simulink model "KLQR"  (R2021b)
settings: Solver=ode23t  StartTime=0.0  StopTime=inf  FixedStep=0.001  RelTol=1e-3
values from neighbouring files (symbols this model uses):
  b = 0.6    [Start.m]
  cf = -54000    [Start.m]
  cr = -54000    [Start.m]
  index_num = length(xr)    [Start.m]
  kappar = refPoses(:,5)'    [Start.m]
  m = 260    [Start.m]
  Pre_kr_num = floor(Pre_distance/d_kr)    [Start.m]
  thetar = refPoses(:,3)'    [Start.m]
  xr = refPoses(:,1)'    [Start.m]
  yr = refPoses(:,2)'    [Start.m]
libraries: vehdynlibviscommon x2, autolibshared x2, mpclib x1
settings Model: Creator=HS  LastModifiedBy=Administrator
settings SolverCC: AlgebraicLoopSolver=TrustRegion
settings OptimizationCC: DefaultParameterBehavior=Inlined  UseDivisionForNetSlopeComputation=on  GainParamInheritBuiltInType=on  UseFloatMulNetSlope=on  InlineInvariantSignals=on  PassReuseOutputArgsAs=Individual arguments  ZeroExternalMemoryAtStartup=off  ZeroInternalMemoryAtStartup=off  NoFixptDivByZeroProtection=on  EfficientFloat2IntCast=on  LifeSpan=1  OptimizeBlockOrder=speed  DifferentSizesBufferReuse=on  EfficientTunableParamExpr=on
settings DebuggingCC: ParameterTunabilityLossMsg=error  SFMachineParentedDataDiag=warning
settings HardwareCC: ProdBitPerLong=64  ProdLongLongMode=on  ProdHWDeviceType=Intel->x86-64 (Linux 64)
settings SFSimCC: MATLABDynamicMemAlloc=off
settings RTWCC: Description=Embedded Coder  SystemTargetFile=ert.tlc  GenCodeOnly=on  TemplateMakefile=ert_default_tmf  GenerateReport=on  IncludeHyperlinkInReport=on  LaunchReport=on  GenerateTraceInfo=on  GenerateTraceReport=on  GenerateTraceReportSl=on  GenerateTraceReportSf=on  GenerateTraceReportEml=on  GenerateCodeMetricsReport=on
settings CodeAppCC: ForceParamTrailComments=on  IgnoreCustomStorageClasses=off  OperatorAnnotations=on  SimulinkDataObjDesc=on  SFDataObjDesc=on  CustomSymbolStrGlobalVar=rt$N$M  CustomSymbolStrType=$N$M  CustomSymbolStrFcn=$N$M$F  CustomSymbolStrMacro=$N$M  InsertBlockDesc=on
settings ERTTargetCC: TargetLangStandard=C99 (ISO)  GenerateSampleERTMain=on  IncludeMdlTerminateFcn=off  CombineSignalStateStructs=on  SupportAbsoluteTime=off  SupportComplex=off  SupportNonInlinedSFcns=on  InlinedParameterPlacement=NonHierarchical  ERTCustomFileTemplate=example_file_process.tlc  ERTFilePackagingFormat=CompactWithDataFile

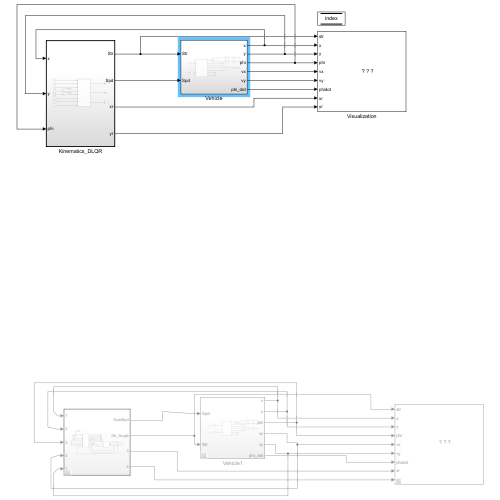
[thumbnail: Simulink's stored preview of the top-level diagram]
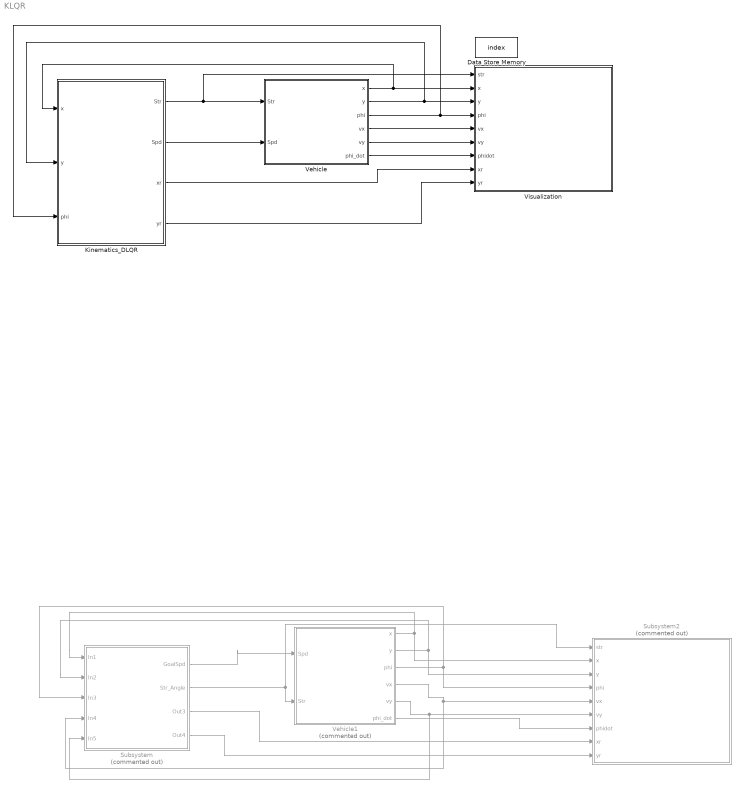
== system KLQR ==
  Data Store Memory : DataStoreMemory  DataStoreName=index  ReadBeforeWriteMsg=warning  WriteAfterWriteMsg=warning  WriteAfterReadMsg=warning  ShowAdditionalParam=off  OutDataTypeStr=double
  Kinematics_DLQR : Subsystem  TreatAsAtomicUnit=on  SystemSampleTime=0.01
  Subsystem : Subsystem  Commented=on  TreatAsAtomicUnit=on  SystemSampleTime=0.01
  Subsystem2 : Subsystem  Commented=on
      mask Display: image('C:\Users\HS\Desktop\Path_Track\Pic\visualization.JPG'); % Use "Edit Image" on toolstrip to change.
  Vehicle : Subsystem
  Vehicle1 : Subsystem  Commented=on
  Visualization : Subsystem
      mask Display: image('C:\Users\HS\Desktop\Path_Track\Pic\visualization.JPG'); % Use "Edit Image" on toolstrip to change.
  wires:
  Kinematics_DLQR/3(xr) -> Visualization/8(xr)
  Kinematics_DLQR/4(yr) -> Visualization/9(yr)
  Kinematics_DLQR/1(Str) -> Visualization/1(str), Vehicle/1(Str)
  Kinematics_DLQR/2(Spd) -> Vehicle/2(Spd)
  Vehicle/1(x) -> Kinematics_DLQR/1(x), Visualization/2(x)
  Vehicle/4(vx) -> Visualization/5(vx)
  Vehicle/5(vy) -> Visualization/6(vy)
  Vehicle/2(y) -> Visualization/3(y), Kinematics_DLQR/2(y)
  Vehicle/6(phi_dot) -> Visualization/7(phidot)
  Vehicle/3(phi) -> Visualization/4(phi), Kinematics_DLQR/3(phi)
  Vehicle1/3(phi) -> Subsystem2/4(phi), Subsystem/3(In3)
  Vehicle1/4(vx) -> Subsystem/4(In4), Subsystem2/5(vx)
  Vehicle1/5(vy) -> Subsystem/5(In5), Subsystem2/6(vy)
  Vehicle1/1(x) -> Subsystem2/2(x), Subsystem/1(In1)
  Vehicle1/2(y) -> Subsystem2/3(y), Subsystem/2(In2)
  Vehicle1/6(phi_dot) -> Subsystem2/7(phidot)
  Subsystem/2(Str_Angle) -> Subsystem2/1(str), Vehicle1/2(Str)
  Subsystem/1(GoalSpd) -> Vehicle1/1(Spd)
  Subsystem/3(Out3) -> Subsystem2/8(xr)
  Subsystem/4(Out4) -> Subsystem2/9(yr)

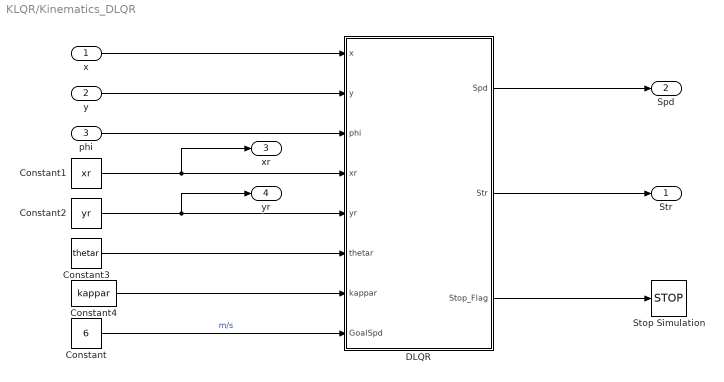
== system KLQR/Kinematics_DLQR ==
  x : Inport
  y : Inport  Port=2
  phi : Inport  Port=3
  Constant : Constant  Value=6
  Constant1 : Constant  Value=xr
  Constant2 : Constant  Value=yr
  Constant3 : Constant  Value=thetar
  Constant4 : Constant  Value=kappar
  DLQR : MATLAB Function  TreatAsAtomicUnit=on
  Stop Simulation : Stop
  Str : Outport
  Spd : Outport  Port=2
  xr : Outport  Port=3
  yr : Outport  Port=4
  wires:
  Constant2/1 -> yr/1, DLQR/5(yr)
  DLQR/3(Stop_Flag) -> Stop Simulation/1
  y/1 -> DLQR/2(y)
  Constant/1 -> DLQR/8(GoalSpd)  "m/s"
  DLQR/2(Str) -> Str/1
  Constant4/1 -> DLQR/7(kappar)
  Constant1/1 -> DLQR/4(xr), xr/1
  Constant3/1 -> DLQR/6(thetar)
  x/1 -> DLQR/1(x)
  DLQR/1(Spd) -> Spd/1
  phi/1 -> DLQR/3(phi)

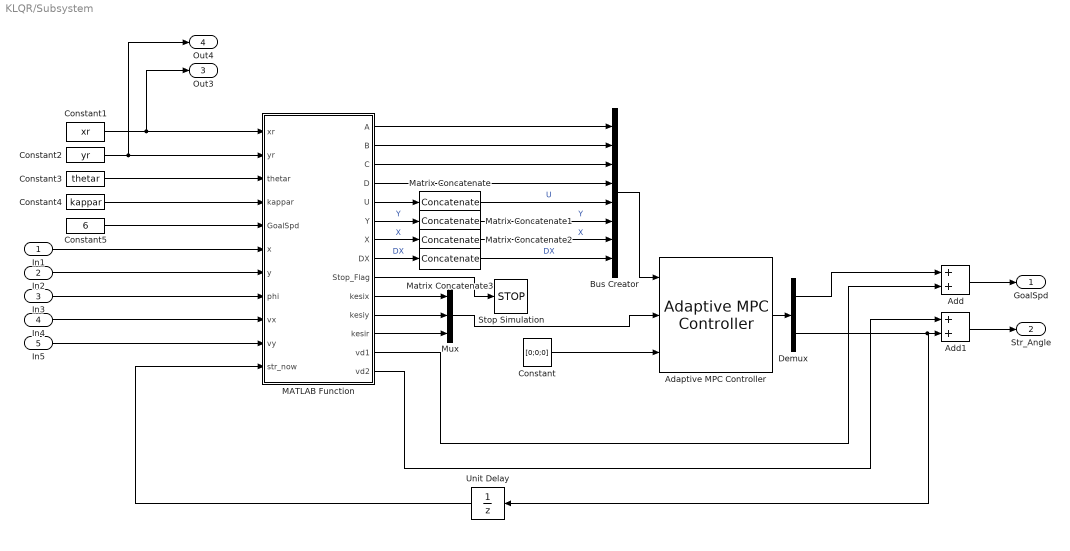
== system KLQR/Subsystem ==
  In1 : Inport
  In2 : Inport  Port=2
  In3 : Inport  Port=3
  In4 : Inport  Port=4
  In5 : Inport  Port=5
  Adaptive MPC Controller : mpclib/Adaptive MPC Controller  SCDEnableBlockLinearizationSpecification=on  mpcobj=mpcobj  enable_value=0  updateMPCinCallerWorkspace=on  md_inport=off  mv_inport=off  uref_inport=off  return_cost=off  return_mvseq=off  return_qpstatus=off  return_xseq=off  return_state=off  return_ovseq=off  state_inport=off  isltv_plant=off  umin_inport=off  umax_inport=off  ymin_inport=off  ymax_inport=off  cc_inport=off  ywt_inport=off  uwt_inport=off  duwt_inport=off  rhoeps_inport=off  pm_inport=off  MaximumP=10  HorizonChoice=FixedHorizon  BlockDataType=double  SampleTimeInherited=off  switch_inport=off
  Add : Sum
  Add1 : Sum
  Bus Creator : BusCreator  Inputs=8
  Constant : Constant  Value=[0;0;0]
  Constant1 : Constant  Value=xr
  Constant2 : Constant  Value=yr
  Constant3 : Constant  Value=thetar
  Constant4 : Constant  Value=kappar
  Constant5 : Constant  Value=6
  Demux : Demux  Outputs=2
  MATLAB Function : MATLAB Function  TreatAsAtomicUnit=on
  Matrix Concatenate : Concatenate  NumInputs=1  Mode=Multidimensional array  ConcatenateDimension=2
  Matrix Concatenate1 : Concatenate  NumInputs=1  Mode=Multidimensional array  ConcatenateDimension=3
  Matrix Concatenate2 : Concatenate  NumInputs=1  Mode=Multidimensional array  ConcatenateDimension=3
  Matrix Concatenate3 : Concatenate  NumInputs=1  Mode=Multidimensional array  ConcatenateDimension=3
  Mux : Mux  Inputs=3
  Stop Simulation : Stop
  Unit Delay : UnitDelay  SampleTime=-1  HasFrameUpgradeWarning=on
  GoalSpd : Outport
  Str_Angle : Outport  Port=2
  Out3 : Outport  Port=3
  Out4 : Outport  Port=4
  wires:
  MATLAB Function/3(C) -> Bus Creator/3
  MATLAB Function/2(B) -> Bus Creator/2
  Bus Creator/1 -> Adaptive MPC Controller/1
  MATLAB Function/4(D) -> Bus Creator/4
  MATLAB Function/1(A) -> Bus Creator/1
  Constant4/1 -> MATLAB Function/4(kappar)
  Constant/1 -> Adaptive MPC Controller/3
  Adaptive MPC Controller/1 -> Demux/1
  Constant1/1 -> Out3/1, MATLAB Function/1(xr)
  Constant3/1 -> MATLAB Function/3(thetar)
  Constant5/1 -> MATLAB Function/5(GoalSpd)
  MATLAB Function/12(kesir) -> Mux/3
  MATLAB Function/11(kesiy) -> Mux/2
  MATLAB Function/10(kesix) -> Mux/1
  Mux/1 -> Adaptive MPC Controller/2
  Constant2/1 -> Out4/1, MATLAB Function/2(yr)
  MATLAB Function/9(Stop_Flag) -> Stop Simulation/1
  Demux/1 -> Add/1
  In1/1 -> MATLAB Function/6(x)
  In2/1 -> MATLAB Function/7(y)
  In3/1 -> MATLAB Function/8(phi)
  In4/1 -> MATLAB Function/9(vx)
  In5/1 -> MATLAB Function/10(vy)
  Unit Delay/1 -> MATLAB Function/11(str_now)
  MATLAB Function/8(DX) -> Matrix Concatenate3/1  "DX"
  Add/1 -> GoalSpd/1
  Add1/1 -> Str_Angle/1
  Demux/2 -> Unit Delay/1, Add1/2
  MATLAB Function/13(vd1) -> Add/2
  MATLAB Function/14(vd2) -> Add1/1
  MATLAB Function/6(Y) -> Matrix Concatenate1/1  "Y"
  MATLAB Function/7(X) -> Matrix Concatenate2/1  "X"
  MATLAB Function/5(U) -> Matrix Concatenate/1
  Matrix Concatenate/1 -> Bus Creator/5  "U"
  Matrix Concatenate1/1 -> Bus Creator/6  "Y"
  Matrix Concatenate2/1 -> Bus Creator/7  "X"
  Matrix Concatenate3/1 -> Bus Creator/8  "DX"

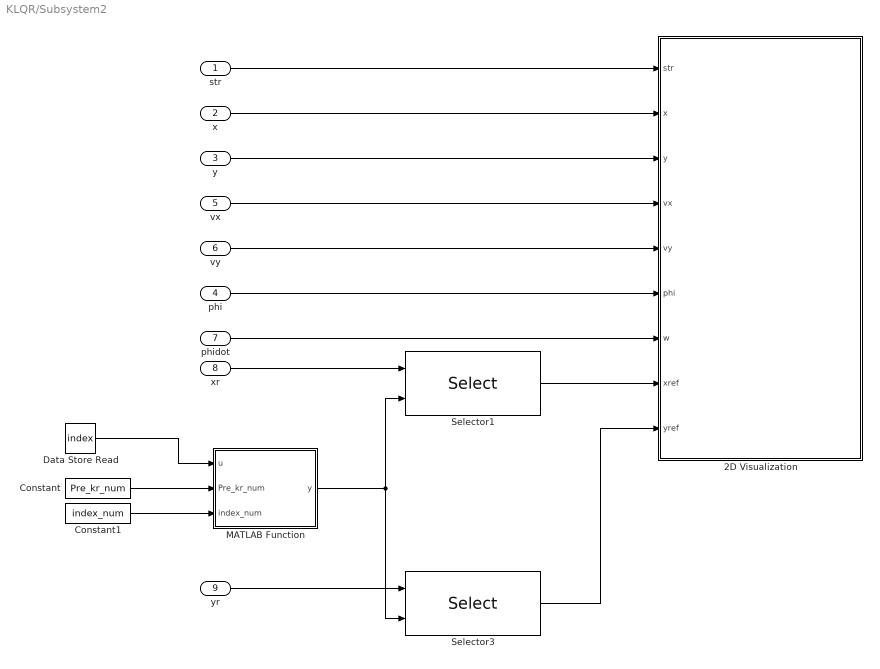
== system KLQR/Subsystem2 ==
  str : Inport
  x : Inport  Port=2
  y : Inport  Port=3
  phi : Inport  Port=4
  vx : Inport  Port=5
  vy : Inport  Port=6
  phidot : Inport  Port=7
  xr : Inport  Port=8
  yr : Inport  Port=9
  2D Visualization : Subsystem
  Constant : Constant  Value=Pre_kr_num
  Constant1 : Constant  Value=index_num
  Data Store Read : DataStoreRead  DataStoreName=index  IndexOptions=Index vector (dialog)  Indices=1  OutputSizes=1
  MATLAB Function : MATLAB Function  TreatAsAtomicUnit=on
  Selector1 : Selector  InputPortWidth=index_num  IndexOptions=Index vector (port)  Indices=[1 3]  OutputSizes=1
  Selector3 : Selector  InputPortWidth=index_num  IndexOptions=Index vector (port)  Indices=[1 3]  OutputSizes=1
  wires:
  Constant1/1 -> MATLAB Function/3(index_num)
  Constant/1 -> MATLAB Function/2(Pre_kr_num)
  MATLAB Function/1(y) -> Selector3/2, Selector1/2
  Data Store Read/1 -> MATLAB Function/1(u)
  str/1 -> 2D Visualization/1(str)
  xr/1 -> Selector1/1
  vy/1 -> 2D Visualization/5(vy)
  x/1 -> 2D Visualization/2(x)
  Selector1/1 -> 2D Visualization/8(xref)
  phidot/1 -> 2D Visualization/7(w)
  phi/1 -> 2D Visualization/6(phi)
  vx/1 -> 2D Visualization/4(vx)
  y/1 -> 2D Visualization/3(y)
  Selector3/1 -> 2D Visualization/9(yref)
  yr/1 -> Selector3/1

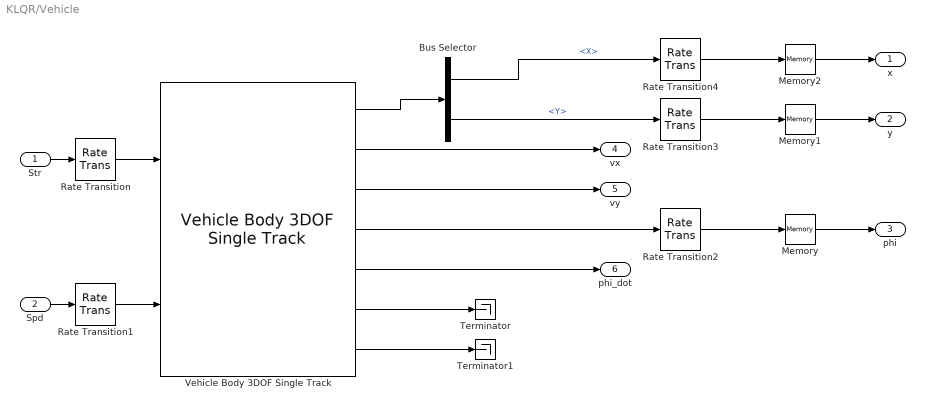
== system KLQR/Vehicle ==
  Str : Inport
  Spd : Inport  Port=2
  Bus Selector : BusSelector  OutputSignals=InertFrm.RearAxl.Disp.X,InertFrm.RearAxl.Disp.Y
  Memory : Memory
  Memory1 : Memory
  Memory2 : Memory
  Rate Transition{,1..4} (5 alike) : RateTransition
  Terminator : Terminator
  Terminator1 : Terminator
  Vehicle Body 3DOF Single Track : autolibshared/Vehicle Body 3DOF Single Track  trackMode=Single (bicycle)  inputMode=External longitudinal velocity  frontSteerMode=on  rearSteerMode=off  windMode=off  muMode=off  extFMode=off  extMMode=off  htchFMode=off  htchMMode=off  extXo=off  extpsio=off  extxdoto=off  extro=off  extYo=off  extTamb=off  extydoto=off  aMode=2  NF=2  NR=2  m=m  a=a  b=b  h=Cg_Height  dh=1  hh=0.2  X_o=xr(1)  xdot_o=0  CalphaMode=off  sigmaMode=off  d=0  hl=0  w=[1.4,1.4]  Cy_f=-cf/2  Cy_r=-cr/2  sigma_f=.1  sigma_r=.1  alpha_f_brk=[-.1 .1]  Cy_f_data=[-9e3 9e3]  alpha_r_brk=[-.1 .1]  Cy_r_data=[-9e3 9e3]  Y_o=yr(1)  ydot_o=0  Izz=Iz  psi_o=thetar(1)  r_o=0  Af=2  Cd=.3  Cl=.1  Cpm=.1  beta_w=[0:0.01:0.3]  Cs=[0:0.03:0.9]  Cym=[0:0.01:0.3]  Pabs=101325  Tair=273  g=9.81  mu=1  xdot_tol=.01  Fznom=5000  Fxtire_sat=7e4  Fytire_sat=7e4  longOff=0  latOff=0  vertOff=0  wrapAng=off
      settings: SourceProductBaseCode=PW,DR,MT,UV,VE
  x : Outport
  y : Outport  Port=2
  phi : Outport  Port=3
  vx : Outport  Port=4
  vy : Outport  Port=5
  phi_dot : Outport  Port=6
  wires:
  Vehicle Body 3DOF Single Track/1 -> Bus Selector/1
  Rate Transition1/1 -> Vehicle Body 3DOF Single Track/2
  Rate Transition4/1 -> Memory2/1
  Rate Transition/1 -> Vehicle Body 3DOF Single Track/1
  Str/1 -> Rate Transition/1
  Bus Selector/2 -> Rate Transition3/1  "<Y>"
  Rate Transition2/1 -> Memory/1
  Rate Transition3/1 -> Memory1/1
  Vehicle Body 3DOF Single Track/4 -> Rate Transition2/1
  Vehicle Body 3DOF Single Track/7 -> Terminator1/1
  Bus Selector/1 -> Rate Transition4/1  "<X>"
  Vehicle Body 3DOF Single Track/6 -> Terminator/1
  Vehicle Body 3DOF Single Track/5 -> phi_dot/1
  Vehicle Body 3DOF Single Track/2 -> vx/1
  Memory/1 -> phi/1
  Memory2/1 -> x/1
  Memory1/1 -> y/1
  Spd/1 -> Rate Transition1/1
  Vehicle Body 3DOF Single Track/3 -> vy/1

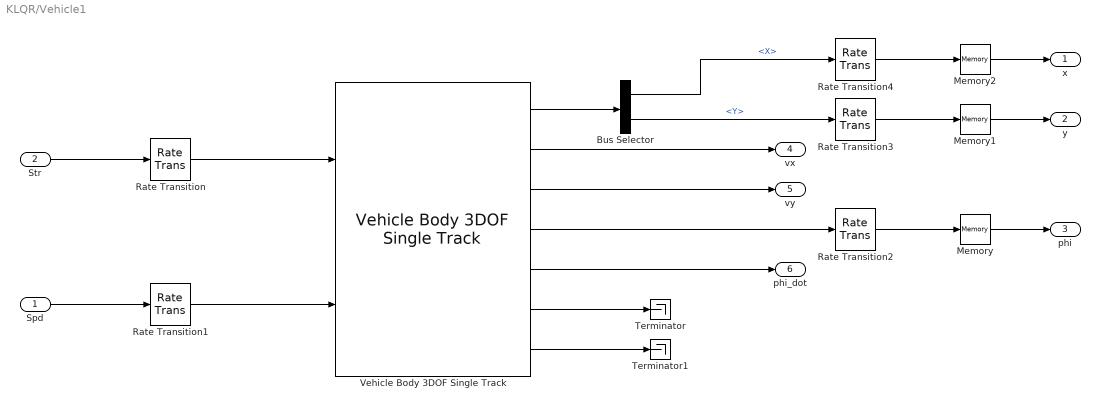
== system KLQR/Vehicle1 ==
  Spd : Inport
  Str : Inport  Port=2
  Bus Selector : BusSelector  OutputSignals=InertFrm.RearAxl.Disp.X,InertFrm.RearAxl.Disp.Y
  Memory : Memory
  Memory1 : Memory
  Memory2 : Memory
  Rate Transition{,1..4} (5 alike) : RateTransition
  Terminator : Terminator
  Terminator1 : Terminator
  Vehicle Body 3DOF Single Track : autolibshared/Vehicle Body 3DOF Single Track  trackMode=Single (bicycle)  inputMode=External longitudinal velocity  frontSteerMode=on  rearSteerMode=off  windMode=off  muMode=off  extFMode=off  extMMode=off  extXo=off  extpsio=off  extxdoto=off  extro=off  extYo=off  extTamb=off  extydoto=off  aMode=2  NF=2  NR=2  m=m  a=a  b=b  h=Cg_Height  X_o=xr(1)  xdot_o=0  CalphaMode=off  sigmaMode=off  d=0  w=[1.4,1.4]  Cy_f=-cf/2  Cy_r=-cr/2  sigma_f=.1  sigma_r=.1  alpha_f_brk=[-.1 .1]  Cy_f_data=[-9e3 9e3]  alpha_r_brk=[-.1 .1]  Cy_r_data=[-9e3 9e3]  Y_o=yr(1)  ydot_o=0  Izz=Iz  psi_o=thetar(1)  r_o=0  Af=2  Cd=.3  Cl=.1  Cpm=.1  beta_w=[0:0.01:0.3]  Cs=[0:0.03:0.9]  Cym=[0:0.01:0.3]  Pabs=101325  Tair=273  g=9.81  mu=1  xdot_tol=.01  Fznom=5000  Fxtire_sat=7e4  Fytire_sat=7e4  longOff=0  latOff=0  vertOff=0  wrapAng=off
      settings: SourceProductBaseCode=PW,DR,MT,UV,VE
  x : Outport
  y : Outport  Port=2
  phi : Outport  Port=3
  vx : Outport  Port=4
  vy : Outport  Port=5
  phi_dot : Outport  Port=6
  wires:
  Vehicle Body 3DOF Single Track/1 -> Bus Selector/1
  Rate Transition1/1 -> Vehicle Body 3DOF Single Track/2
  Rate Transition4/1 -> Memory2/1
  Rate Transition/1 -> Vehicle Body 3DOF Single Track/1
  Str/1 -> Rate Transition/1
  Bus Selector/2 -> Rate Transition3/1  "<Y>"
  Rate Transition2/1 -> Memory/1
  Rate Transition3/1 -> Memory1/1
  Vehicle Body 3DOF Single Track/4 -> Rate Transition2/1
  Vehicle Body 3DOF Single Track/7 -> Terminator1/1
  Bus Selector/1 -> Rate Transition4/1  "<X>"
  Vehicle Body 3DOF Single Track/6 -> Terminator/1
  Vehicle Body 3DOF Single Track/5 -> phi_dot/1
  Vehicle Body 3DOF Single Track/2 -> vx/1
  Memory/1 -> phi/1
  Memory2/1 -> x/1
  Memory1/1 -> y/1
  Spd/1 -> Rate Transition1/1
  Vehicle Body 3DOF Single Track/3 -> vy/1

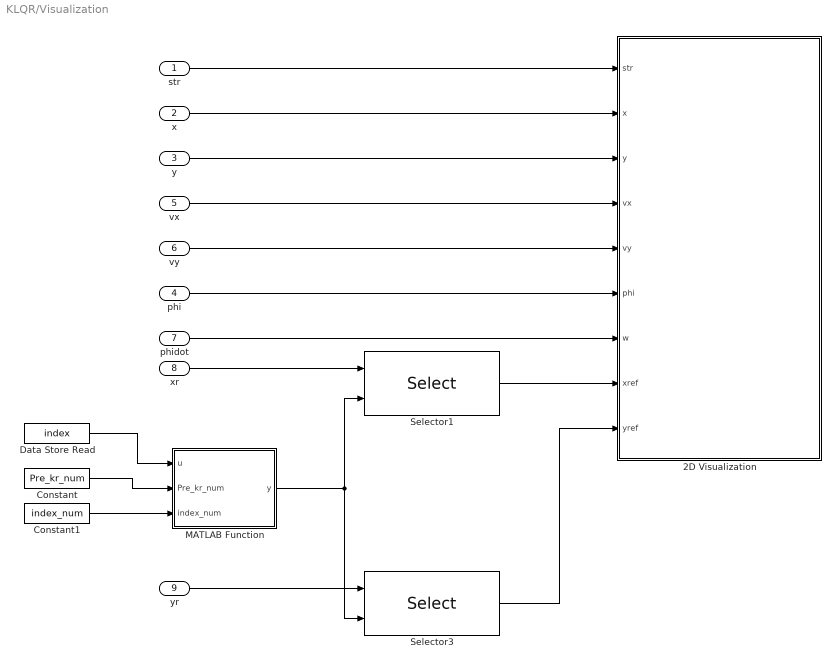
== system KLQR/Visualization ==
  str : Inport
  x : Inport  Port=2
  y : Inport  Port=3
  phi : Inport  Port=4
  vx : Inport  Port=5
  vy : Inport  Port=6
  phidot : Inport  Port=7
  xr : Inport  Port=8
  yr : Inport  Port=9
  2D Visualization : Subsystem
  Constant : Constant  Value=Pre_kr_num
  Constant1 : Constant  Value=index_num
  Data Store Read : DataStoreRead  DataStoreName=index  IndexOptions=Index vector (dialog)  Indices=1  OutputSizes=1
  MATLAB Function : MATLAB Function  TreatAsAtomicUnit=on
  Selector1 : Selector  InputPortWidth=index_num  IndexOptions=Index vector (port)  Indices=[1 3]  OutputSizes=1
  Selector3 : Selector  InputPortWidth=index_num  IndexOptions=Index vector (port)  Indices=[1 3]  OutputSizes=1
  wires:
  yr/1 -> Selector3/1
  Selector3/1 -> 2D Visualization/9(yref)
  y/1 -> 2D Visualization/3(y)
  vx/1 -> 2D Visualization/4(vx)
  phi/1 -> 2D Visualization/6(phi)
  phidot/1 -> 2D Visualization/7(w)
  Selector1/1 -> 2D Visualization/8(xref)
  x/1 -> 2D Visualization/2(x)
  vy/1 -> 2D Visualization/5(vy)
  xr/1 -> Selector1/1
  str/1 -> 2D Visualization/1(str)
  Data Store Read/1 -> MATLAB Function/1(u)
  MATLAB Function/1(y) -> Selector1/2, Selector3/2
  Constant/1 -> MATLAB Function/2(Pre_kr_num)
  Constant1/1 -> MATLAB Function/3(index_num)

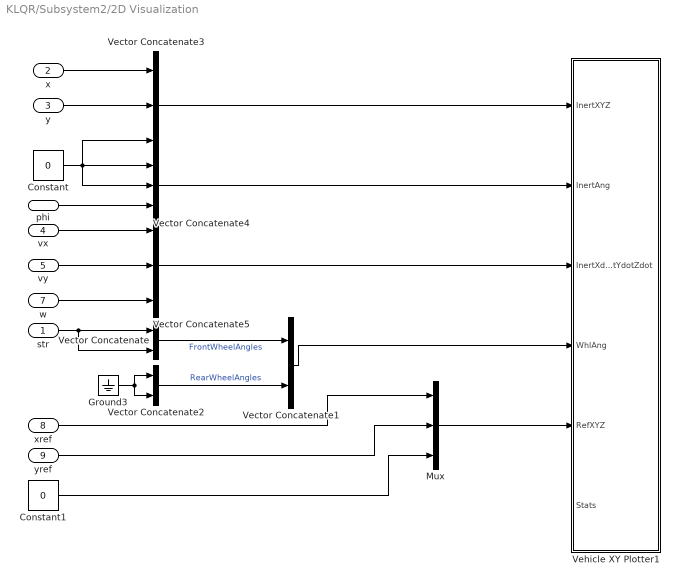
== system KLQR/Subsystem2/2D Visualization ==
  str : Inport
  x : Inport  Port=2
  y : Inport  Port=3
  vx : Inport  Port=4
  vy : Inport  Port=5
  phi : Inport  Port=6
  w : Inport  Port=7
  xref : Inport  Port=8
  yref : Inport  Port=9
  Constant : Constant  Value=0
  Constant1 : Constant  Value=0
  Ground3 : Ground
  Mux : Mux  Inputs=3
  Vector Concatenate : Concatenate
  Vector Concatenate1 : Concatenate
  Vector Concatenate2 : Concatenate
  Vector Concatenate3 : Concatenate  NumInputs=3
  Vector Concatenate4 : Concatenate  NumInputs=3
  Vector Concatenate5 : Concatenate  NumInputs=3
  Vehicle XY Plotter1 : Subsystem  mask(Vehicle XY Plotter){extRef=on, extStats=on, extTireF=off, a=1, b=0.6, w=1.49, figBorder=20, bufferSize=1024, velNorm=2, tireFNorm=1000, pltDT=0.05}
      mask prompts: extRef "Plot path reference, extRef"; extStats "Display speed, RPM and Gear"; extTireF "Display tire forces"; a "Distance to front axle from CG, a [m]:"; b "Distance to rear axle from CG, b [m]:"; w "Track width, w [m]:"; figBorder "Distance to figure borders, figBorder [m]:"; bufferSize "Path buffer sampe size, bufferSize []:"; velNorm "Velocity vector scaling, velNorm [m*s/m]:"; tireFNorm "Tire force vector scaling, tireFNorm [m/N]:"; pltDT "Plot update rate, pltDT [s]:"
      mask help:
      | This block will display a MATLAB figure which indicates the vehicle path, current position and heading velocity.
      | An optional path reference is also provided.
      mask init:
      | block = gcb;
      | if autoblkschecksimstopped(block)
      |     ParamNames = {'extRef';'extStats';'extTireF';'extTireF'};
      |     PortNames = {'RefXYZ';'Stats';'TireFx';'TireFy'};
      |     for idx=1:length(PortNames)
      |         InportOption  = {'built-in/Ground', [PortNames{idx}, ' Ground'];...
      |             'built-in/Inport',PortNames{idx}};
      |         if ~strcmp(get_param(block,ParamNames{idx}),'on')
      |             NewBlkHdl = autoblksreplaceblock(block, InportOption, 1);
      |             set_param(NewBlkHdl, 'ShowName', 'off');
      |         else
      |             autoblksreplaceblock(block, InportOption, 2);
      |         end
      |     end
      |     InportNames = {'InertXYZ';'InertAng';'InertXdotYdotZdot';'WhlAng';'RefXYZ';'Stats';'TireFx';'TireFy'};
      |     FoundNames = get_param(find_system(block, 'LookUnderMasks', 'all', 'SearchDepth', 1, 'FollowLinks', 'on', 'BlockType', 'Inport'), 'Name');
      |     [~,PortI] = intersect(InportNames, FoundNames);
      |     PortI = sort(PortI);
      |     for idx = 1:length(PortI)
      |         set_param([block, '/', InportNames{PortI(idx)}], 'Port', num2str(idx));
      |     end
      | end
      mask TypeOptions a: Vehicle XY Plotter/a
      mask TypeOptions b: Vehicle XY Plotter/b
      mask TypeOptions w: Vehicle XY Plotter/w
      mask TypeOptions figBorder: Vehicle XY Plotter/figBorder
      mask TypeOptions bufferSize: Vehicle XY Plotter/bufferSize
      mask TypeOptions velNorm: Vehicle XY Plotter/velNorm
      mask TypeOptions tireFNorm: Vehicle XY Plotter/tireFNorm
      mask DialogControl Container3 Prompt: Plot and Display Options
  wires:
  phi/1 -> Vector Concatenate4/3
  Constant1/1 -> Mux/3
  yref/1 -> Mux/2
  xref/1 -> Mux/1
  Mux/1 -> Vehicle XY Plotter1/5(RefXYZ)
  str/1 -> Vector Concatenate/1, Vector Concatenate/2
  vx/1 -> Vector Concatenate5/1
  w/1 -> Vector Concatenate5/3
  vy/1 -> Vector Concatenate5/2
  Constant/1 -> Vector Concatenate4/2, Vector Concatenate4/1, Vector Concatenate3/3
  y/1 -> Vector Concatenate3/2
  x/1 -> Vector Concatenate3/1
  Vector Concatenate4/1 -> Vehicle XY Plotter1/2(InertAng)
  Vector Concatenate3/1 -> Vehicle XY Plotter1/1(InertXYZ)
  Vector Concatenate5/1 -> Vehicle XY Plotter1/3(InertXdotYdotZdot)
  Vector Concatenate2/1 -> Vector Concatenate1/2  "RearWheelAngles"
  Vector Concatenate/1 -> Vector Concatenate1/1  "FrontWheelAngles"
  Ground3/1 -> Vector Concatenate2/2, Vector Concatenate2/1
  Vector Concatenate1/1 -> Vehicle XY Plotter1/4(WhlAng)

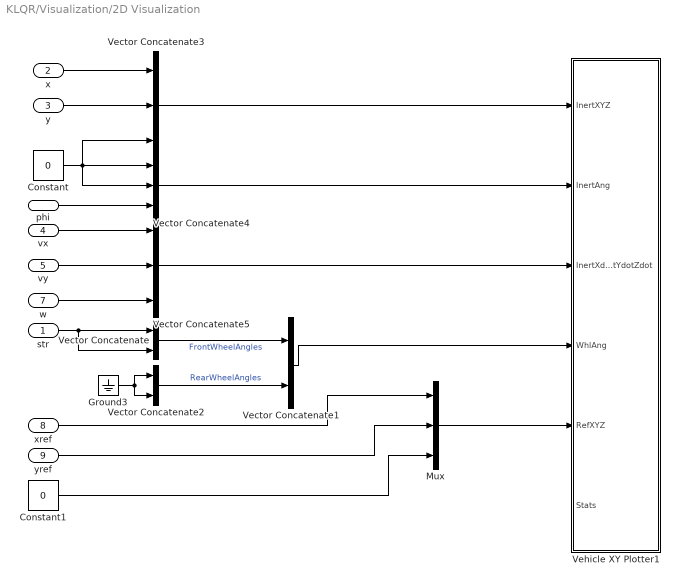
== system KLQR/Visualization/2D Visualization ==
  str : Inport
  x : Inport  Port=2
  y : Inport  Port=3
  vx : Inport  Port=4
  vy : Inport  Port=5
  phi : Inport  Port=6
  w : Inport  Port=7
  xref : Inport  Port=8
  yref : Inport  Port=9
  Constant : Constant  Value=0
  Constant1 : Constant  Value=0
  Ground3 : Ground
  Mux : Mux  Inputs=3
  Vector Concatenate : Concatenate
  Vector Concatenate1 : Concatenate
  Vector Concatenate2 : Concatenate
  Vector Concatenate3 : Concatenate  NumInputs=3
  Vector Concatenate4 : Concatenate  NumInputs=3
  Vector Concatenate5 : Concatenate  NumInputs=3
  Vehicle XY Plotter1 : Subsystem  mask(Vehicle XY Plotter){extRef=on, extStats=on, extTireF=off, a=1, b=0.6, w=1.49, figBorder=20, bufferSize=1024, velNorm=2, tireFNorm=1000, pltDT=0.05}
      mask prompts: extRef "Plot path reference, extRef"; extStats "Display speed, RPM and Gear"; extTireF "Display tire forces"; a "Distance to front axle from CG, a [m]:"; b "Distance to rear axle from CG, b [m]:"; w "Track width, w [m]:"; figBorder "Distance to figure borders, figBorder [m]:"; bufferSize "Path buffer sampe size, bufferSize []:"; velNorm "Velocity vector scaling, velNorm [m*s/m]:"; tireFNorm "Tire force vector scaling, tireFNorm [m/N]:"; pltDT "Plot update rate, pltDT [s]:"
      mask help:
      | This block will display a MATLAB figure which indicates the vehicle path, current position and heading velocity.
      | An optional path reference is also provided.
      mask init: same as KLQR/Subsystem2/2D Visualization/Vehicle XY Plotter1
      mask TypeOptions a: Vehicle XY Plotter/a
      mask TypeOptions b: Vehicle XY Plotter/b
      mask TypeOptions w: Vehicle XY Plotter/w
      mask TypeOptions figBorder: Vehicle XY Plotter/figBorder
      mask TypeOptions bufferSize: Vehicle XY Plotter/bufferSize
      mask TypeOptions velNorm: Vehicle XY Plotter/velNorm
      mask TypeOptions tireFNorm: Vehicle XY Plotter/tireFNorm
      mask DialogControl Container3 Prompt: Plot and Display Options
  wires:
  Vector Concatenate1/1 -> Vehicle XY Plotter1/4(WhlAng)
  Ground3/1 -> Vector Concatenate2/1, Vector Concatenate2/2
  Vector Concatenate/1 -> Vector Concatenate1/1  "FrontWheelAngles"
  Vector Concatenate2/1 -> Vector Concatenate1/2  "RearWheelAngles"
  Vector Concatenate5/1 -> Vehicle XY Plotter1/3(InertXdotYdotZdot)
  Vector Concatenate3/1 -> Vehicle XY Plotter1/1(InertXYZ)
  Vector Concatenate4/1 -> Vehicle XY Plotter1/2(InertAng)
  x/1 -> Vector Concatenate3/1
  y/1 -> Vector Concatenate3/2
  Constant/1 -> Vector Concatenate3/3, Vector Concatenate4/1, Vector Concatenate4/2
  vy/1 -> Vector Concatenate5/2
  w/1 -> Vector Concatenate5/3
  vx/1 -> Vector Concatenate5/1
  str/1 -> Vector Concatenate/2, Vector Concatenate/1
  Mux/1 -> Vehicle XY Plotter1/5(RefXYZ)
  xref/1 -> Mux/1
  yref/1 -> Mux/2
  Constant1/1 -> Mux/3
  phi/1 -> Vector Concatenate4/3

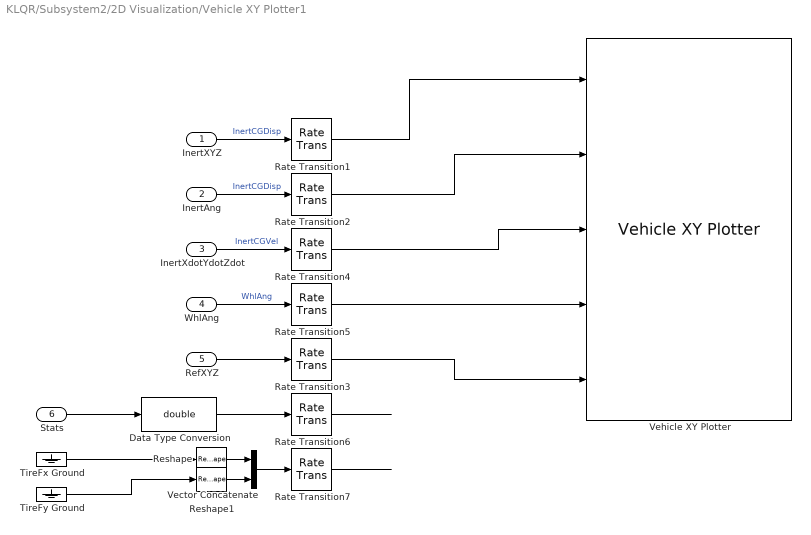
== system KLQR/Subsystem2/2D Visualization/Vehicle XY Plotter1 ==
  InertXYZ : Inport
  InertAng : Inport  Port=2
  InertXdotYdotZdot : Inport  Port=3
  WhlAng : Inport  Port=4
  RefXYZ : Inport  Port=5
  Stats : Inport  Port=6
  Data Type Conversion : DataTypeConversion  OutDataTypeStr=double
  Rate Transition{1..7} (7 alike) : RateTransition  Deterministic=off  OutPortSampleTime=pltDT
  Reshape : Reshape  OutputDimensionality=Row vector (2-D)
  Reshape1 : Reshape  OutputDimensionality=Row vector (2-D)
  TireFx Ground : Ground
  TireFy Ground : Ground
  Vector Concatenate : Concatenate  Mode=Multidimensional array
  Vehicle XY Plotter : vehdynlibviscommon/Vehicle XY Plotter  w=w  a=a  b=b  figBorder=figBorder  bufferSize=bufferSize  extStats=off  extTireF=off
      settings: SourceProductBaseCode=VE
  wires:
  Stats/1 -> Data Type Conversion/1
  TireFy Ground/1 -> Reshape1/1
  TireFx Ground/1 -> Reshape/1
  InertAng/1 -> Rate Transition2/1  "InertCGDisp"
  InertXdotYdotZdot/1 -> Rate Transition4/1  "InertCGVel"
  InertXYZ/1 -> Rate Transition1/1  "InertCGDisp"
  WhlAng/1 -> Rate Transition5/1  "WhlAng"
  Rate Transition3/1 -> Vehicle XY Plotter/5
  Rate Transition1/1 -> Vehicle XY Plotter/1
  Rate Transition2/1 -> Vehicle XY Plotter/2
  Rate Transition4/1 -> Vehicle XY Plotter/3
  Rate Transition5/1 -> Vehicle XY Plotter/4
  Rate Transition6/1 -> ?
  Data Type Conversion/1 -> Rate Transition6/1
  Rate Transition7/1 -> ?
  RefXYZ/1 -> Rate Transition3/1
  Reshape/1 -> Vector Concatenate/1
  Reshape1/1 -> Vector Concatenate/2
  Vector Concatenate/1 -> Rate Transition7/1

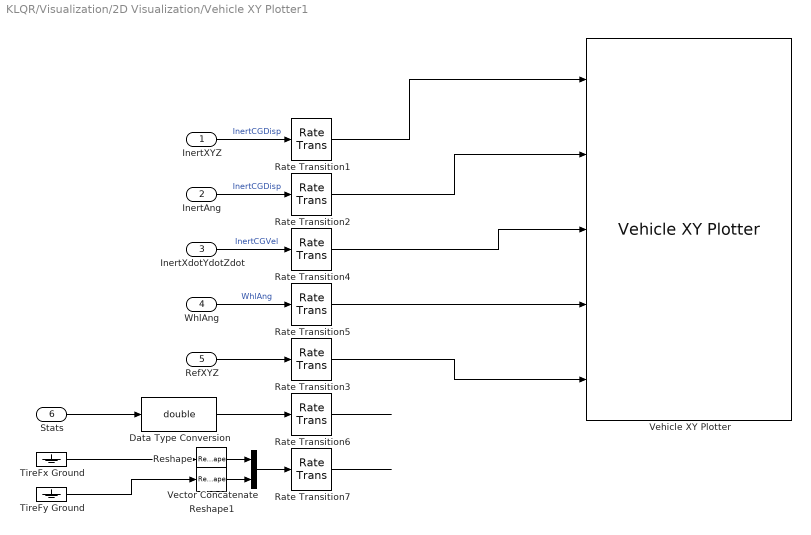
== system KLQR/Visualization/2D Visualization/Vehicle XY Plotter1 ==
  InertXYZ : Inport
  InertAng : Inport  Port=2
  InertXdotYdotZdot : Inport  Port=3
  WhlAng : Inport  Port=4
  RefXYZ : Inport  Port=5
  Stats : Inport  Port=6
  Data Type Conversion : DataTypeConversion  OutDataTypeStr=double
  Rate Transition{1..7} (7 alike) : RateTransition  Deterministic=off  OutPortSampleTime=pltDT
  Reshape : Reshape  OutputDimensionality=Row vector (2-D)
  Reshape1 : Reshape  OutputDimensionality=Row vector (2-D)
  TireFx Ground : Ground
  TireFy Ground : Ground
  Vector Concatenate : Concatenate  Mode=Multidimensional array
  Vehicle XY Plotter : vehdynlibviscommon/Vehicle XY Plotter  w=w  a=a  b=b  figBorder=figBorder  bufferSize=bufferSize  extStats=off  extTireF=off
      settings: SourceProductBaseCode=VE
  wires:
  Vector Concatenate/1 -> Rate Transition7/1
  Reshape1/1 -> Vector Concatenate/2
  Reshape/1 -> Vector Concatenate/1
  RefXYZ/1 -> Rate Transition3/1
  Rate Transition7/1 -> ?
  Data Type Conversion/1 -> Rate Transition6/1
  Rate Transition6/1 -> ?
  Rate Transition5/1 -> Vehicle XY Plotter/4
  Rate Transition4/1 -> Vehicle XY Plotter/3
  Rate Transition2/1 -> Vehicle XY Plotter/2
  Rate Transition1/1 -> Vehicle XY Plotter/1
  Rate Transition3/1 -> Vehicle XY Plotter/5
  WhlAng/1 -> Rate Transition5/1  "WhlAng"
  InertXYZ/1 -> Rate Transition1/1  "InertCGDisp"
  InertXdotYdotZdot/1 -> Rate Transition4/1  "InertCGVel"
  InertAng/1 -> Rate Transition2/1  "InertCGDisp"
  TireFx Ground/1 -> Reshape/1
  TireFy Ground/1 -> Reshape1/1
  Stats/1 -> Data Type Conversion/1

== matlab function KLQR/Subsystem2/MATLAB Function ==
  data: u input; Pre_kr_num input; index_num input; y output
function y = fcn(u, Pre_kr_num, index_num)

if u + Pre_kr_num*8 < index_num
    y = u + Pre_kr_num*8;
else
    y = index_num;
end

end

== matlab function KLQR/Subsystem/MATLAB Function ==
  data: xr input; A output; yr input; thetar input; kappar input; GoalSpd input; x input; y input; phi input; vx input; vy input; str_now input; B output; C output; D output; U output; Y output; X output; DX output; Stop_Flag output; kesix output; kesiy output; kesir output; index data_store_memory; vd1 output; vd2 output
function [A,B,C,D,U,Y,X,DX,Stop_Flag,kesix,kesiy,kesir,vd1,vd2] = fcn(xr,yr,thetar,kappar,GoalSpd,x,y,phi,vx,vy,str_now)
%****初始化参数矩阵************%
global index;
T = 0.01;%程序离散控制周期，配合原子子系统0.01ms周期
L = 1.6;%车辆轴距
n=length(xr);      %路径点个数
Stop_Flag = 0;     %仿真结束标志位
%coder.extrinsic('dlqr'); %若用自带库函数，请用外部声明
min=1;
%*******寻找车辆后轴与当前车辆最近点，仅查找距上一次车辆位置最近点前30个点
    if index == 0  %%Code has not run yet;
		d_min=(x-xr(1))^2+(y-yr(1))^2;
		min=1;
		for i=1:30 %% search 1-30 points when car is running.
			d=(x-xr(i))^2+(y-yr(i))^2;
			if d<d_min
				d_min=d;
				min=i;
			end
		end
		dmin=min;
		index = dmin; %% dmin assigns to index;
    else
		d_min = (x-xr(index))^2+(y-yr(index))^2;
		min = index;
		if index <= n - 30
			for i = index:index+30
				d=(x-xr(i))^2+(y-yr(i))^2;
				if d<d_min
					d_min=d;
					min=i;
				end
			end
			dmin=min;
			index = dmin;
		else 
			for i = index:n
				d=(x-xr(i))^2+(y-yr(i))^2;
				if d<d_min
					d_min=d;
					min=i;
                    if min == n
                        Stop_Flag =1;%路径点跑完了仿真停止
                    end
				end
			end
			dmin=min;
			index = dmin; 
		end
    end
%*****状态变量计算******%
kesix = x -xr(dmin);
kesiy = y -yr(dmin);
kesir =phi - thetar(dmin);
  %******防止数据溢出***********%
    if kesir < -3.14
        kesir = kesir+6.28;
    end
    if kesir >3.14
        kesir = kesir -6.28;
    end
xstate = [kesix;
          kesiy;
          kesir];%状态变量
vd1 = GoalSpd; %期望速度
t_d = thetar(dmin);%当前和车辆最近点的航向角
k = kappar(dmin);%当前和车辆最近点的曲率
vd2=atan(L*k);%期望前轮转角
Ad=[1    0   -vd1*sin(t_d)*T;
    0    1   vd1*cos(t_d)*T;
    0    0    1;];  %线性离散后的系统矩阵   
Bd=[cos(t_d)*T     0;
    sin(t_d)*T     0;
    tan(vd2)*T/L   vd1*T/(L*(cos(vd2)^2))]; %线性离散后的控制矩阵
Cd =[1 0 0;
    0 1 0;
    0 0 1;];
Dd = [0 0 ; 0  0;0  0];
A =Ad;
B =Bd;
C =Cd;
D =Dd;
X = xstate;
v_now =sqrt(vx^2+vy^2);
U = [vd1 - v_now;
    vd2 - str_now];
Y =C*xstate;
DX = A*xstate+B*U-xstate;





end

== matlab function KLQR/Visualization/MATLAB Function ==
  data: u input; Pre_kr_num input; index_num input; y output
function y = fcn(u, Pre_kr_num, index_num)

if u + Pre_kr_num*8 < index_num
    y = u + Pre_kr_num*8;
else
    y = index_num;
end

end

== matlab function KLQR/Kinematics_DLQR/DLQR ==
  settings: updateMethod=DISCRETE
  data: Spd output; Str output; x input; y input; phi input; xr input; yr input; thetar input; kappar input; Stop_Flag output; index data_store_memory; GoalSpd input

function [Spd,Str,Stop_Flag]  = fcn(x,y,phi,xr,yr,thetar,kappar,GoalSpd)
%****初始化参数矩阵************%
global index;
T = 0.01;%程序离散控制周期，配合原子子系统0.01ms周期
L = 1.6;%车辆轴距
PN_1 = zeros(3,3); %该矩阵用于黎卡提方程迭代
n=length(xr);      %路径点个数
Stop_Flag = 0;     %仿真结束标志位
I = eye(3);        %初始化3*3单位矩阵
K =zeros(2,3);     %初始化反馈增益矩阵维度
%coder.extrinsic('dlqr'); %若用自带库函数，请用外部声明
min=1;
%*******寻找车辆后轴与当前车辆最近点，仅查找距上一次车辆位置最近点前30个点
    if index == 0  %%Code has not run yet;
		d_min=(x-xr(1))^2+(y-yr(1))^2;
		min=1;
		for i=1:30 %% search 1-30 points when car is running.
			d=(x-xr(i))^2+(y-yr(i))^2;
			if d<d_min
				d_min=d;
				min=i;
			end
		end
		dmin=min;
		index = dmin; %% dmin assigns to index;
    else
		d_min = (x-xr(index))^2+(y-yr(index))^2;
		min = index;
		if index <= n - 30
			for i = index:index+30
				d=(x-xr(i))^2+(y-yr(i))^2;
				if d<d_min
					d_min=d;
					min=i;
				end
			end
			dmin=min;
			index = dmin;
		else 
			for i = index:n
				d=(x-xr(i))^2+(y-yr(i))^2;
				if d<d_min
					d_min=d;
					min=i;
                    if min == n
                        Stop_Flag =1;%路径点跑完了仿真停止
                    end
				end
			end
			dmin=min;
			index = dmin; 
		end
    end
%*****状态变量计算******%
kesix = x -xr(dmin);
kesiy = y -yr(dmin);
kesir =phi - thetar(dmin);
  %******防止偏差数据溢出***********%
    if kesir < -3.14
        kesir = kesir+6.28;
    end
    if kesir >3.14
        kesir = kesir -6.28;
    end

xstate = [kesix;
          kesiy;
          kesir];%状态变量
vd1 = GoalSpd; %期望速度
t_d = thetar(dmin);%当前和车辆最近点的航向角
k = kappar(dmin);%当前和车辆最近点的曲率
vd2=atan(L*k);%期望前轮转角

Ad=[1    0   -vd1*sin(t_d)*T;
    0    1   vd1*cos(t_d)*T;
    0    0    1;];  %线性离散后的系统矩阵
   
Bd=[cos(t_d)*T     0;
    sin(t_d)*T     0;
    tan(vd2)*T/L   vd1*T/(L*(cos(vd2)^2))]; %线性离散后的控制矩阵
   
 Q = [10 0 0;
      0 10 0; 
      0 0 10];%初始化LQR的权重矩阵
 R =[5 0;
     0 5];%初始化LQR的权重矩阵
 
 %*********黎卡提方程求解**********%
 PN =Q;  
 err =10^(-1);%该精度根据需要调整，误差越小迭代次数越多
 error = 1;
 while(error>err)
        PN_1 = Q+Ad'*PN/(I+Bd/R*Bd'*PN)*Ad;%黎卡提方程
        error = norm(PN-PN_1);
        PN =PN_1;
        i = i+1;%观察迭代步数
        if i>40000 %防止迭代次数过长，该值根据控制器实际性能设置
            break;
        end
 end
 P =PN_1;
 K = (R+Bd'*P*Bd)\Bd'*P*Ad;%计算状态反馈增益K
  %***************************************%
  
%K =dlqr(Ad,Bd,Q,R); %使用官方求解库，配合外部函数引用才有效，否则报错。
 U  = - K * xstate; %线性反馈控制量
 deltav = U(1);
 deltastr =U(2);
 
 Spd = GoalSpd+deltav; %m/s
 Str = vd2+deltastr; %rad
end
